simulink model "dpsk_N3"  (R2020b)
settings: Solver=VariableStepAuto  StartTime=0.0  StopTime=stopTime  RelTol=1e-3
values from neighbouring files (symbols this model uses):
  indexMat = reshape(preIndexMat, 2, M^2)    [dpsk_N3_parameters.m]
  M = 8    [dpsk_N3_parameters.m]
undefined symbols (not defined in the file or in its folder): mainMat
libraries: commchan3 x1, commsink2 x1, commdigbbndpm3 x1, commrandsrc3 x1
settings Model: Creator=Peyton  LastModifiedBy=Peyton

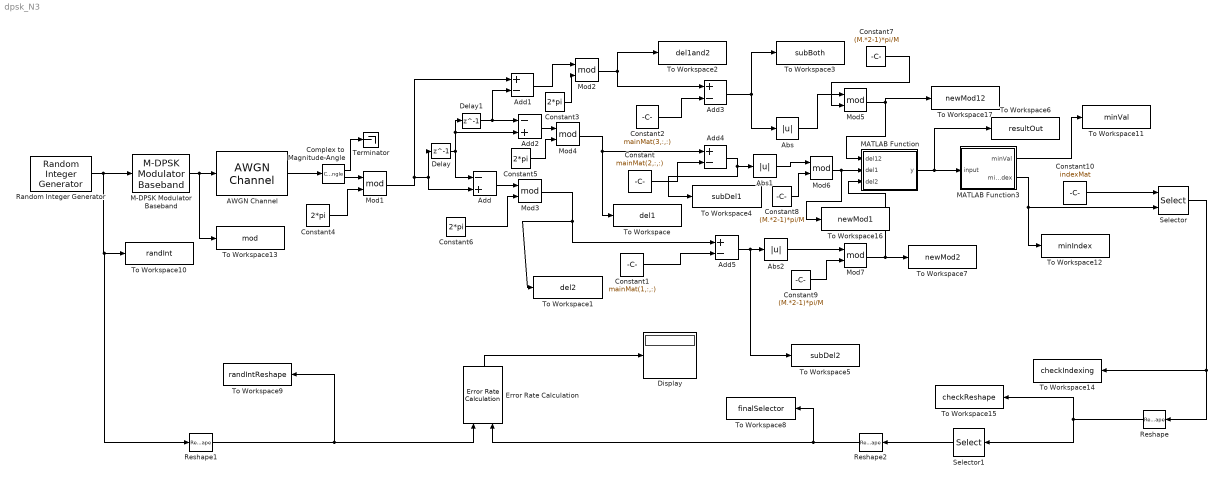
== system dpsk_N3 ==
  AWGN Channel : commchan3/AWGN Channel  InputProcessing=Columns as channels (frame based)  seed=67  noiseMode="Signal to noise ratio  (Eb/No)"  EbNodB=snr  EsNodB=10  SNRdB=10  bitsPerSym=log2(M)  Ps=1  Tsym=1  variance=1
  Abs : Abs
  Abs1 : Abs
  Abs2 : Abs
  Add : Sum  Inputs=-+
  Add{1,3..5} (4 alike) : Sum  Inputs=+-
  Add2 : Sum  Inputs=-+
  Complex to Magnitude-Angle : ComplexToMagnitudeAngle
  Constant : Constant  Value=mainMat(2,:,:)
  Constant1 : Constant  Value=mainMat(1,:,:)
  Constant10 : Constant  Value=indexMat
  Constant2 : Constant  Value=mainMat(3,:,:)
  Constant{3..6} (4 alike) : Constant  Value=2*pi
  Constant7 : Constant  Value=(M.*2-1)*pi/M
  Constant8 : Constant  Value=(M.*2-1)*pi/M
  Constant9 : Constant  Value=(M.*2-1)*pi/M
  Delay : Delay  DelayLength=1  InitialCondition=0
  Delay1 : Delay  DelayLength=1  InitialCondition=0
  Display : Display
  Error Rate Calculation : commsink2/Error Rate Calculation  N=0  st_delay=0  cp_mode=Entire frame  subframe=[]  PMode=Port  WsName=ErrorVec  RsMode2=off  stop=off  numErr=100  maxBits=1e6
      settings: SourceProductName=Communications Toolbox
  M-DPSK Modulator Baseband : commdigbbndpm3/M-DPSK Modulator Baseband  M=M  InType=Integer  Enc=Binary  Ph=0  outDtype=double
      settings: SourceProductBaseCode=CM
  MATLAB Function : MATLAB Function  TreatAsAtomicUnit=on
  MATLAB Function3 : MATLAB Function  TreatAsAtomicUnit=on
  Mod{1..7} (7 alike) : Math  Operator=mod  SaturateOnIntegerOverflow=on
  Random Integer Generator : commrandsrc3/Random Integer Generator  SetSize=M  SeedSource=Auto  Seed=0  SampleTime=1  SamplesPerFrame=1  OutputDataType=double  SimulateUsing=Interpreted execution
  Reshape : Reshape
  Reshape1 : Reshape
  Reshape2 : Reshape
  Selector : Selector  NumberOfDimensions=2  InputPortWidth=3  IndexOptions=Select all,Index vector (port)  Indices=[1 3],1  OutputSizes=1,1
  Selector1 : Selector  NumberOfDimensions=2  InputPortWidth=3  IndexOptions=Select all,Index vector (dialog)  Indices=[1 3],1  OutputSizes=1,1
  Terminator : Terminator
  To Workspace : ToWorkspace  VariableName=del1  SampleTime=-1
  To Workspace1 : ToWorkspace  VariableName=del2  SampleTime=-1
  To Workspace10 : ToWorkspace  VariableName=randInt  SampleTime=-1
  To Workspace11 : ToWorkspace  VariableName=minVal  SampleTime=-1
  To Workspace12 : ToWorkspace  VariableName=minIndex  SampleTime=-1
  To Workspace13 : ToWorkspace  VariableName=mod  SampleTime=-1
  To Workspace14 : ToWorkspace  VariableName=checkIndexing  SampleTime=-1
  To Workspace15 : ToWorkspace  VariableName=checkReshape  SampleTime=-1
  To Workspace16 : ToWorkspace  VariableName=newMod1  SampleTime=-1
  To Workspace17 : ToWorkspace  VariableName=newMod12  SampleTime=-1
  To Workspace2 : ToWorkspace  VariableName=del1and2  SampleTime=-1
  To Workspace3 : ToWorkspace  VariableName=subBoth  SampleTime=-1
  To Workspace4 : ToWorkspace  VariableName=subDel1  SampleTime=-1
  To Workspace5 : ToWorkspace  VariableName=subDel2  SampleTime=-1
  To Workspace6 : ToWorkspace  VariableName=resultOut  SampleTime=-1
  To Workspace7 : ToWorkspace  VariableName=newMod2  SampleTime=-1
  To Workspace8 : ToWorkspace  VariableName=finalSelector  SampleTime=-1
  To Workspace9 : ToWorkspace  VariableName=randIntReshape  SampleTime=-1
  wires:
  Random Integer Generator/1 -> Reshape1/1, To Workspace10/1, M-DPSK Modulator Baseband/1
  M-DPSK Modulator Baseband/1 -> To Workspace13/1, AWGN Channel/1
  AWGN Channel/1 -> Complex to Magnitude-Angle/1
  Complex to Magnitude-Angle/1 -> Terminator/1
  Complex to Magnitude-Angle/2 -> Mod1/1
  Mod1/1 -> Add1/1, Delay/1, Add/2
  Delay/1 -> Add2/2, Delay1/1, Add/1
  Delay1/1 -> Add1/2, Add2/1
  Add1/1 -> Mod2/1
  Mod2/1 -> To Workspace2/1, Add3/1
  Add/1 -> Mod3/1
  Mod3/1 -> Add5/1, To Workspace1/1
  Add2/1 -> Mod4/1
  Mod4/1 -> Add4/1, To Workspace/1
  Constant/1 -> Add4/2
  Constant2/1 -> Add3/2
  Constant1/1 -> Add5/2
  Add3/1 -> Abs/1, To Workspace3/1
  MATLAB Function/1(y) -> To Workspace6/1, MATLAB Function3/1(input)
  Constant4/1 -> Mod1/2
  Constant3/1 -> Mod2/2
  Constant6/1 -> Mod3/2
  Constant5/1 -> Mod4/2
  Add4/1 -> To Workspace4/1, Abs1/1
  Add5/1 -> To Workspace5/1, Abs2/1
  MATLAB Function3/1(minVal) -> To Workspace11/1
  MATLAB Function3/2(minIndex) -> Selector/2, To Workspace12/1
  Constant10/1 -> Selector/1
  Selector/1 -> Reshape/1, To Workspace14/1
  Reshape/1 -> To Workspace15/1, Selector1/1
  Reshape1/1 -> To Workspace9/1, Error Rate Calculation/1
  Selector1/1 -> Reshape2/1
  Error Rate Calculation/1 -> Display/1
  Reshape2/1 -> Error Rate Calculation/2, To Workspace8/1
  Abs/1 -> Mod5/1
  Constant7/1 -> Mod5/2
  Mod5/1 -> MATLAB Function/1(del12), To Workspace17/1
  Abs1/1 -> Mod6/1
  Abs2/1 -> Mod7/1
  Constant9/1 -> Mod7/2
  Constant8/1 -> Mod6/2
  Mod6/1 -> To Workspace16/1, MATLAB Function/2(del1)
  Mod7/1 -> To Workspace7/1, MATLAB Function/3(del2)

== matlab function dpsk_N3/MATLAB Function ==
  data: del12 input; y output; del1 input; del2 input
function y = fcn(del12, del1,del2)

y = abs(del2(:,:,:,:) + del1(:,:,:,:) + del12(:,:,:,:));

== matlab function dpsk_N3/MATLAB Function3 ==
  data: input input; minVal output; minIndex output
function [minVal, minIndex] = fcn(input)

[minVal, minIndex] = min(input, [], [1 2 3], 'linear');
